simulink model "RST_PresSim_R2013b"  (R2022b)
settings: Solver=FixedStepDiscrete  StartTime=0.0  StopTime=0.001*84*0+inf  FixedStep=0.05  RelTol=1e-3
values from neighbouring files (symbols this model uses):
  Am = H_0dt.den{1}    [VariantaBUNA10.m]
  Bm = H_0dt.num{1}    [VariantaBUNA10.m]
  S = conv(S1, [1, -1])    [VariantaBUNA10.m]
  T = H0d.den{1}/ sum(B)    [VariantaBUNA10.m]
undefined symbols (not defined in the file or in its folder): R
libraries: instrumentlib x2
settings Model: Creator=Severus  LastModifiedBy=saioc
settings SolverCC: AlgebraicLoopSolver=TrustRegion
settings DataIOCC: SaveFormat=StructureWithTime  ReturnWorkspaceOutputs=off
settings OptimizationCC: LifeSpan=inf
settings DebuggingCC: UnconnectedInputMsg=warning  UnconnectedOutputMsg=warning  UnconnectedLineMsg=warning  SFExecutionAtInitializationDiag=none  SFMachineParentedDataDiag=warning  ArithmeticOperatorsInVariantConditions=warning
settings HardwareCC: ProdBitPerSizeT=32  ProdBitPerPtrDiffT=32  ProdWordSize=32  ProdHWDeviceType=Specified
settings SFSimCC: SimUseLocalCustomCode=off  CustomCodeUndefinedFunction=UseInterfaceOnly
settings RTWCC: RTWUseLocalCustomCode=off  RTWCompilerOptimization=on
settings CodeAppCC: MaxIdLength=95  StateflowObjectComments=on

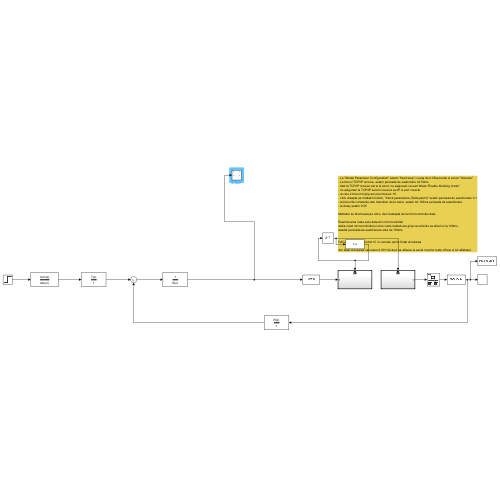
[thumbnail: Simulink's stored preview of the top-level diagram]
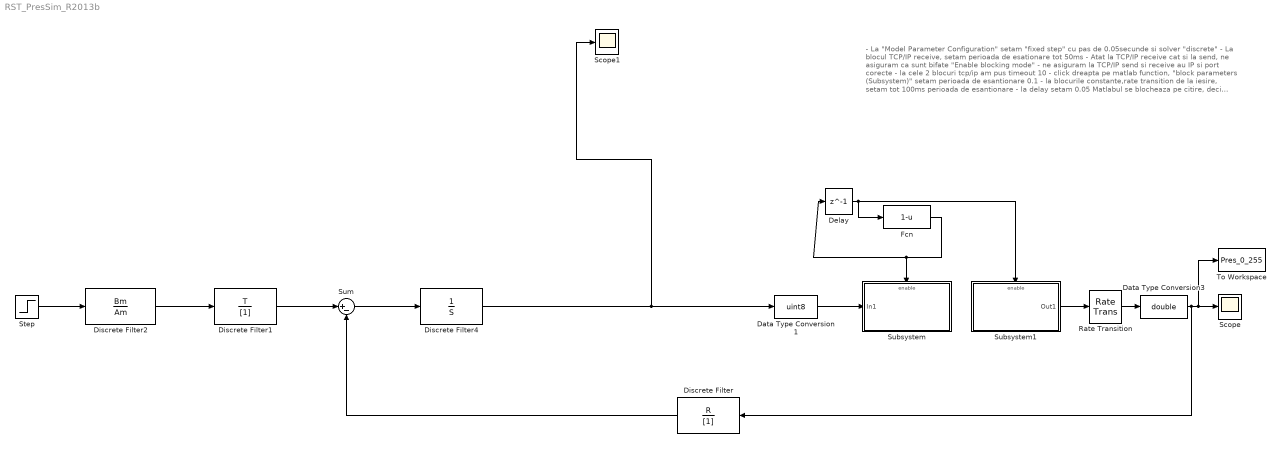
== system RST_PresSim_R2013b ==
  note: - La "Model Parameter Configuration" setam "fixed step" cu pas de 0.05secunde si solver "discrete"
      | - La blocul TCP/IP receive, setam perioada de esationare tot 50ms
      | - Atat la TCP/IP receive cat si la send, ne asiguram ca sunt bifate "Enable blocking mode"
      | - ne asiguram la TCP/IP send si receive au IP si port corecte
      | - la cele 2 blocuri tcp/ip am pus timeout 10
      | - click dreapta pe matlab function, "block parameters (Subsystem)" setam perioada de esantionare 0.1
      | - la blocurile constante,rate transition de la iesire, setam tot 100ms perioada de esantionare
      | - la delay setam 0.05
      |
      | Matlabul se blocheaza pe citire, deci asteapta de la microcontroller date
      |
      | Esantionarea reala este data din microcontroller
      | adica cand microcontrollerul scrie catre matlab are grija ca scrierile sa aiba loc la 100ms
      | asadar perioada de esantionare este de 100ms
      |
      |
      | DACA da eroare, Control+C in consola oprim fortat simularea
      |
      | Am lasat simularea sa ruleze 0.001*42 deci sa afiseze la serial monitor toate cifrele si tot alfabetul
  Data Type Conversion1 : DataTypeConversion  OutDataTypeStr=uint8  SaturateOnIntegerOverflow=off  RndMeth=Floor
  Data Type Conversion3 : DataTypeConversion  OutDataTypeStr=double  SaturateOnIntegerOverflow=off  RndMeth=Floor
  Delay : Delay  DelayLength=1  InitialCondition=0  SampleTime=0.05
  Discrete Filter : DiscreteFilter  Numerator=R  Denominator=[1]  SampleTime=0.1
  Discrete Filter1 : DiscreteFilter  Numerator=T  Denominator=[1]  SampleTime=0.1
  Discrete Filter2 : DiscreteFilter  Numerator=Bm  Denominator=Am  SampleTime=0.1
  Discrete Filter4 : DiscreteFilter  Numerator=1  Denominator=S  SampleTime=0.1
  Fcn : Fcn  Expr=1-u
  Rate Transition : RateTransition  OutPortSampleTime=0.1
  Scope : Scope
  Scope1 : Scope
  Step : Step  Time=0  After=100  SampleTime=0.1
  Subsystem : Subsystem
  Subsystem1 : Subsystem
  Sum : Sum  Inputs=|+-
  To Workspace : ToWorkspace  VariableName=Pres_0_255  SaveFormat=Timeseries  SampleTime=-1
  wires:
  Sum/1 -> Discrete Filter4/1
  Subsystem1/1(Out1) -> Rate Transition/1
  Delay/1 -> Subsystem1/Enable, Fcn/1
  Rate Transition/1 -> Data Type Conversion3/1
  Data Type Conversion1/1 -> Subsystem/1(In1)
  Fcn/1 -> Subsystem/Enable, Delay/1
  Data Type Conversion3/1 -> Discrete Filter/1, To Workspace/1, Scope/1
  Discrete Filter4/1 -> Scope1/1, Data Type Conversion1/1
  Discrete Filter/1 -> Sum/2
  Discrete Filter2/1 -> Discrete Filter1/1
  Discrete Filter1/1 -> Sum/1
  Step/1 -> Discrete Filter2/1

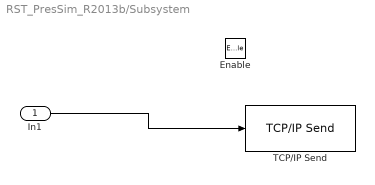
== system RST_PresSim_R2013b/Subsystem ==
  In1 : Inport
  Enable : EnablePort
  TCP/IP Send : instrumentlib/TCP//IP Send  Host=192.168.0.103  Port=94  ByteOrder=big-endian  EnableBlockingMode=on  Timeout=10  TransferDelay=on  SimulateUsing=Interpreted execution
  wires:
  In1/1 -> TCP/IP Send/1

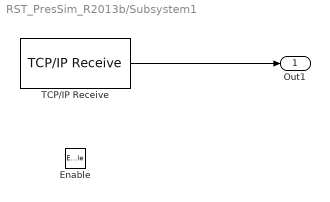
== system RST_PresSim_R2013b/Subsystem1 ==
  Enable : EnablePort
  TCP/IP Receive : instrumentlib/TCP//IP Receive  Host=192.168.0.103  Port=94  DataSize=1  DataType=uint8  ASCIIFormatting=%f  Terminator=LF  CustomTerminator=10  ByteOrder=big-endian  EnableBlockingMode=on  Timeout=10  SampleTime=0.05  SimulateUsing=Interpreted execution
  Out1 : Outport
  wires:
  TCP/IP Receive/1 -> Out1/1
